simulink model "battery_hybrid_digital_twin"  (R2023b)
settings: Solver=FixedStepDiscrete  StartTime=0.0  StopTime=inf  FixedStep=1  RelTol=1e-3
libraries: simulink x9
settings Model: Creator=SREEKAR  LastModifiedBy=SREEKAR

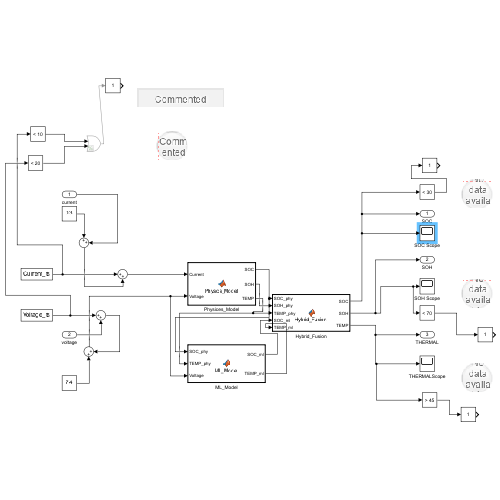
[thumbnail: Simulink's stored preview of the top-level diagram]
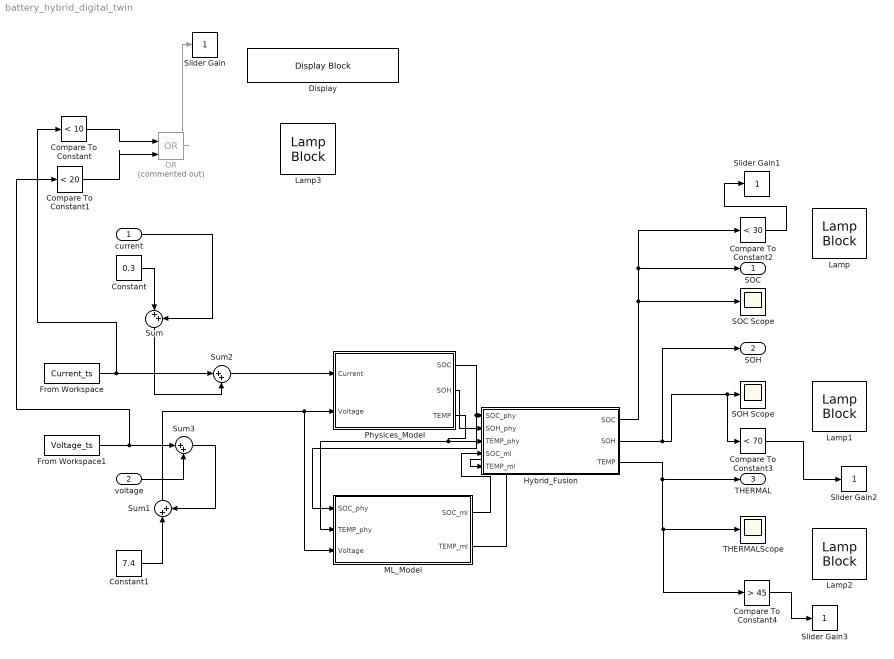
== system battery_hybrid_digital_twin ==
  current : Inport
  voltage : Inport  Port=2
  Compare To Constant : simulink/Logic and Bit Operations/Compare To Constant  relop=<  const=10  OutDataTypeStr=boolean
  Compare To Constant1 : simulink/Logic and Bit Operations/Compare To Constant  relop=<  const=20  OutDataTypeStr=boolean
  Compare To Constant2 : simulink/Logic and Bit Operations/Compare To Constant  relop=<  const=30  OutDataTypeStr=boolean
  Compare To Constant3 : simulink/Logic and Bit Operations/Compare To Constant  relop=<  const=70  OutDataTypeStr=boolean
  Compare To Constant4 : simulink/Logic and Bit Operations/Compare To Constant  relop=>  const=45  OutDataTypeStr=boolean
  Constant : Constant  Value=0.3
  Constant1 : Constant  Value=7.4
  Display : DisplayBlock  LabelPosition=Hide  Transparency=1
  From Workspace : FromWorkspace  VariableName=Current_ts  SampleTime=1
  From Workspace1 : FromWorkspace  VariableName=Voltage_ts  SampleTime=1
  Hybrid_Fusion : MATLAB Function  TreatAsAtomicUnit=on
  Lamp{,1..3} (4 alike) : LampBlock  LabelPosition=Hide
  ML_Model : MATLAB Function  TreatAsAtomicUnit=on
  OR : Logic  Commented=on  Operator=OR  IconShape=distinctive  AllPortsSameDT=off  OutDataTypeStr=boolean
  Physices_Model : MATLAB Function  TreatAsAtomicUnit=on
  SOC Scope : Scope
  SOH Scope : Scope
  Slider Gain{,1..3} (4 alike) : simulink/Math Operations/Slider Gain  gain=1  low=0  high=2
  Sum{,1..3} (4 alike) : Sum  Inputs=|++
  THERMALScope : Scope
  SOC : Outport
  SOH : Outport  Port=2
  THERMAL : Outport  Port=3
  wires:
  Physices_Model/1(SOC) -> Hybrid_Fusion/1(SOC_phy), ML_Model/1(SOC_phy)
  Physices_Model/2(SOH) -> Hybrid_Fusion/2(SOH_phy)
  Physices_Model/3(TEMP) -> ML_Model/2(TEMP_phy), Hybrid_Fusion/3(TEMP_phy)
  ML_Model/1(SOC_ml) -> Hybrid_Fusion/4(SOC_ml)
  ML_Model/2(TEMP_ml) -> Hybrid_Fusion/5(TEMP_ml)
  Hybrid_Fusion/1(SOC) -> Compare To Constant2/1, SOC/1, SOC Scope/1
  Hybrid_Fusion/3(TEMP) -> Compare To Constant4/1, THERMALScope/1, THERMAL/1
  Hybrid_Fusion/2(SOH) -> SOH/1, Compare To Constant3/1, SOH Scope/1
  Constant/1 -> Sum/1
  Constant1/1 -> Sum1/1
  voltage/1 -> Sum3/2
  Sum1/1 -> ML_Model/3(Voltage), Physices_Model/2(Voltage)
  From Workspace/1 -> Compare To Constant/1, Sum2/1
  From Workspace1/1 -> Compare To Constant1/1, Sum3/1
  Sum3/1 -> Sum1/2
  current/1 -> Sum/2
  Sum/1 -> Sum2/2
  Sum2/1 -> Physices_Model/1(Current)
  Compare To Constant/1 -> OR/1
  Compare To Constant1/1 -> OR/2
  OR/1 -> Slider Gain/1
  Compare To Constant2/1 -> Slider Gain1/1
  Compare To Constant3/1 -> Slider Gain2/1
  Compare To Constant4/1 -> Slider Gain3/1

== matlab function battery_hybrid_digital_twin/ML_Model ==
  data: SOC_phy input; SOC_ml output; TEMP_phy input; Voltage input; TEMP_ml output
function [SOC_ml, TEMP_ml] = ML_Model(SOC_phy, TEMP_phy, Voltage)
% Lightweight ML Model (Data-driven approximation)
% SAFE version – all outputs assigned

% ---------- DEFAULT OUTPUT ASSIGNMENT ----------
SOC_ml  = 0;
TEMP_ml = 0;

% ---------- SIMPLE DATA-DRIVEN LOGIC ----------
% (Proxy ML model – extend later if needed)

SOC_ml  = SOC_phy;
TEMP_ml = TEMP_phy;
TEMP_ml = TEMP_phy + 0.01 * (Voltage - 7.4);

== matlab function battery_hybrid_digital_twin/Physices_Model ==
  data: Current input; SOC output; SOH output; TEMP output; Voltage input
function [SOC, SOH, TEMP] = Physics_Model(Current, Voltage)
% Battery Physics Digital Twin
% SAFE version – all outputs assigned on all paths

% ---------- DEFAULT OUTPUT ASSIGNMENT (VERY IMPORTANT) ----------
SOC  = 0;
SOH  = 0;
TEMP = 0;

% ---------- PERSISTENT STATES ----------
persistent soc_prev soh_prev
if isempty(soc_prev)
    soc_prev = 100;   % initial SOC (%)
    soh_prev = 100;   % initial SOH (%)
end

% ---------- PARAMETERS ----------
Ts = 1;            % sample time (s)
Capacity = 0.5;    % 500 mAh = 0.5 Ah

% ---------- SOC (Coulomb Counting) ----------
soc_prev = soc_prev - (Current * Ts / 3600) / Capacity * 100;
soc_prev = max(0, min(100, soc_prev));

% ---------- SOH (Simple Degradation) ----------
soh_prev = soh_prev - 0.0005 * abs(Current);
soh_prev = max(0, soh_prev);
% SOH degradation influenced by voltage stress
% SOH degradation influenced by voltage stress
soh_prev = soh_prev - 0.0005 * abs(Current) - 0.0001 * abs(Voltage - 7.4);

% ---------- THERMAL MODEL ----------
TEMP = 25 + (Current^2 * 2.0);

% ---------- FINAL OUTPUT ASSIGNMENT ----------
SOC = soc_prev;
SOH = soh_prev;

== matlab function battery_hybrid_digital_twin/Hybrid_Fusion ==
  data: SOC_phy input; SOC output; SOH_phy input; TEMP_phy input; SOC_ml input; TEMP_ml input; SOH output; TEMP output
function [SOC, SOH, TEMP] = Hybrid_Fusion( ...
    SOC_phy, SOH_phy, TEMP_phy, SOC_ml, TEMP_ml)
% Hybrid Digital Twin Fusion Block
% SAFE version – deterministic outputs

% ---------- DEFAULT OUTPUT ASSIGNMENT ----------
SOC  = 0;
SOH  = 0;
TEMP = 0;

% ---------- FUSION WEIGHTS ----------
w_phy = 0.6;
w_ml  = 0.4;

% ---------- HYBRID FUSION ----------
SOC  = w_phy * SOC_phy  + w_ml * SOC_ml;
SOH  = SOH_phy;                 % ML SOH optional
TEMP = w_phy * TEMP_phy + w_ml * TEMP_ml;
SOC  = 0.6 * SOC_phy + 0.4 * SOC_ml;
SOH  = SOH_phy;
TEMP = 0.5 * TEMP_phy + 0.5 * TEMP_ml;
